simulink model "Lab4_closedloop_speed_control"  (R2016b)
settings: Solver=VariableStepAuto  StartTime=0.0  StopTime=2  RelTol=1e-3  EnableMultiTasking=on
libraries: powerlib x8, simulink x1
settings Model: Creator=Yash Bansod  LastModifiedBy=Yash Bansod
settings DataIOCC: LimitDataPoints=on
settings OptimizationCC: LifeSpan=inf
settings DebuggingCC: AllowSymbolicDim=off  SFUnexpectedBacktrackingDiag=warning  SFNoUnconditionalDefaultTransitionDiag=warning  SFExecutionAtInitializationDiag=none
settings ModelReferenceCC: PropagateSignalLabelsOutOfModel=off
settings GRTTargetCC: TargetLangStandard=C89/C90 (ANSI)
settings ConfigComp: CovMetricSettings=dw  CovHtmlReporting=on  CovSaveCumulativeToWorkspaceVar=on  CovSaveSingleToWorkspaceVar=on  CovExternalEMLEnable=off

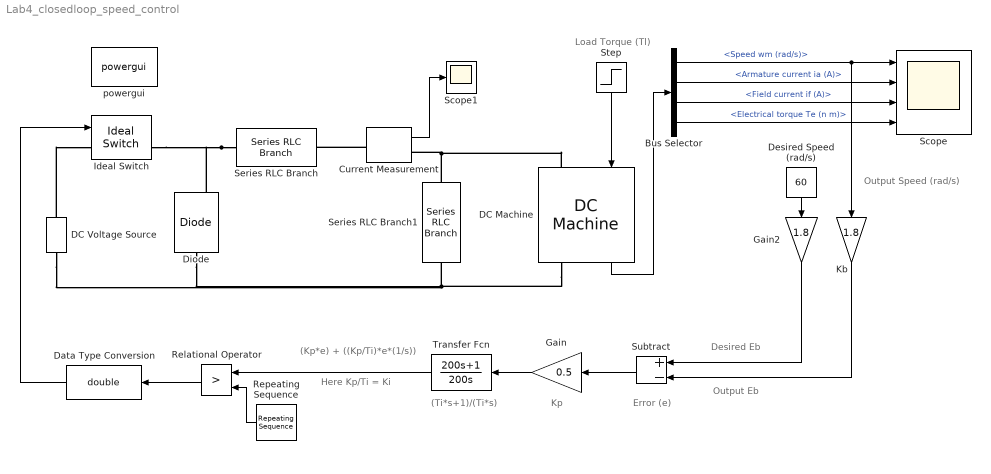
== system Lab4_closedloop_speed_control ==
  note: Load Torque (Tl)
  note: (Kp*e) + ((Kp/Ti)*e*(1/s))
  note: Here Kp/Ti = Ki
  note: (Ti*s+1)/(Ti*s)
  note: Kp
  note: Error (e)
  note: Desired Eb
  note: Output Eb
  note: Output Speed (rad/s)
  Bus Selector : BusSelector  OutputSignals=Speed wm (rad/s),Armature current ia (A),Field current if (A),Electrical torque Te (n m)
  Current Measurement : powerlib/Measurements/Current Measurement  PhasorSimulation=off  OutputType=Complex  PSBequivalent=0
  DC Machine : powerlib/Machines/DC Machine  PresetModel=No  MechanicalLoad=Torque TL  FieldType=Permanent magnet  ShowDetailedParameters=on  MeasurementBus=off  RLa="[ 0.6  0.012]"  RLf="[ 240  120]"  Laf=1.8  MachineConstant=Torque constant (N.m/A)  Ke=1.8  Kt=1.8  J=1  Bm=0  Tf=0  w0=1  Ifinit=1  TsPowergui=0  TsBlock=-1
  DC Voltage Source : powerlib/Electrical Sources/DC Voltage Source  Amplitude=220  Measurements=Voltage
  Data Type Conversion : DataTypeConversion  OutDataTypeStr=double
  Desired Speed (rad/s) : Constant  Value=60
  Diode : powerlib/Power Electronics/Diode  Ron=0.001  Lon=0  Vf=0.8  IC=0  UseSnubber=off  Rs=500  Cs=250e-9  Measurements=on
  Gain : Gain  Gain=0.5
  Gain2 : Gain  Gain=1.8
  Ideal Switch : powerlib/Power Electronics/Ideal Switch  Ron=0.001  Lon=0  IC=0  Rs=1e5  Cs=inf  Measurements=on
  Kb : Gain  Gain=1.8
  Relational Operator : RelationalOperator  Operator=>  OutDataTypeStr=boolean  RndMeth=Nearest
  Repeating Sequence : simulink/Sources/Repeating Sequence  rep_seq_t=[0 0.0002]  rep_seq_y=[0 1]
  Scope : Scope  NumInputPorts=4
  Scope1 : Scope
  Series RLC Branch : powerlib/Elements/Series RLC Branch  LConnTagsString=__new0  RConnTagsString=__new0  BranchType=L  Resistance=1  Inductance=300e-6  SetiL0=off  InitialCurrent=0  Capacitance=1e-6  Setx0=off  InitialVoltage=0  Measurements=None
  Series RLC Branch1 : powerlib/Elements/Series RLC Branch  LConnTagsString=__new0  RConnTagsString=__new0  BranchType=C  Resistance=1  Inductance=1e-3  SetiL0=off  InitialCurrent=0  Capacitance=5e-6  Setx0=off  InitialVoltage=0  Measurements=None
  Step : Step  Time=0  After=20  SampleTime=0
  Subtract : Sum  Inputs=+-
  Transfer Fcn : TransferFcn  Numerator=[200 1]  Denominator=[200 0]
  powergui : powerlib/powergui  Priority=1  SimulationMode=Continuous  SolverType=Tustin/Backward Euler (TBE)  SampleTime=50e-6  frequency=60  SPID=on  DisableSnubberDevices=off  DisableRonSwitches=off  DisableVfSwitches=off  SwTol=0  DisplayEquations=off  Interpol=off  ExternalGateDelay=off  methode=off  Ts=10  FunctionMessages=off  echomessages=off  HookPort=off  EnableUseOfTLC=off  x0status=blocks  frequencyindice=0  Pbase=100e6  ErrMax=1e-4  Iterations=50  UnitsV=kV  UnitsW=MW  buscounter=0  RestoreLinks=warning  ResistiveCurrentMeasurement=off  Frange=[0:2:500]  Ylog=off  Xlog=on  ShowGrid=off  save=off  variable=ZData  structure=0  ZoomFFT=off  StartTime=0.0  cycles=1  DisplayStyle=1  fundamental=60  FreqAxis=off  MaxFrequency=1000  frequencyindicesteady=1  RmsSteady=1  display=off
  wires:
  Current Measurement/1 -> Scope1/1
  Subtract/1 -> Gain/1
  Gain/1 -> Transfer Fcn/1
  Transfer Fcn/1 -> Relational Operator/1
  Repeating Sequence/1 -> Relational Operator/2
  Relational Operator/1 -> Data Type Conversion/1
  Data Type Conversion/1 -> Ideal Switch/1
  Bus Selector/1 -> Kb/1, Scope/1  "<Speed wm (rad/s)>"
  Bus Selector/2 -> Scope/2  "<Armature current ia (A)>"
  Bus Selector/3 -> Scope/3  "<Field current if (A)>"
  Bus Selector/4 -> Scope/4  "<Electrical torque Te (n m)>"
  Kb/1 -> Subtract/2
  Desired Speed (rad/s)/1 -> Gain2/1
  Gain2/1 -> Subtract/1
  Step/1 -> DC Machine/1
  DC Machine/1 -> Bus Selector/1
  connections:
  Series RLC Branch1/LConn1 -- DC Machine/LConn1 -- Current Measurement/RConn1
  DC Voltage Source/LConn1 -- Diode/LConn1 -- DC Machine/RConn1 -- Series RLC Branch1/RConn1
  Series RLC Branch/LConn1 -- Ideal Switch/RConn1 -- Diode/RConn1
  Current Measurement/LConn1 -- Series RLC Branch/RConn1
  DC Voltage Source/RConn1 -- Ideal Switch/LConn1
